simulink subsystem "controllerSSNominalReducedOrderObserver"  (R2024b)
settings: Solver=VariableStepAuto  StartTime=0.0  StopTime=10.0  RelTol=1e-3
values from neighbouring files (symbols this model uses):
  K_stateFB = place(A_c, B_c, p)    [Controller_StateSpaceDigitalController.m]
  Nu = Sol(3, :)    [Controller_StateSpaceDigitalController.m]
  Nx = Sol(1:2, :)    [Controller_StateSpaceDigitalController.m]
settings Model: Creator=Utente  LastModifiedBy=Utente

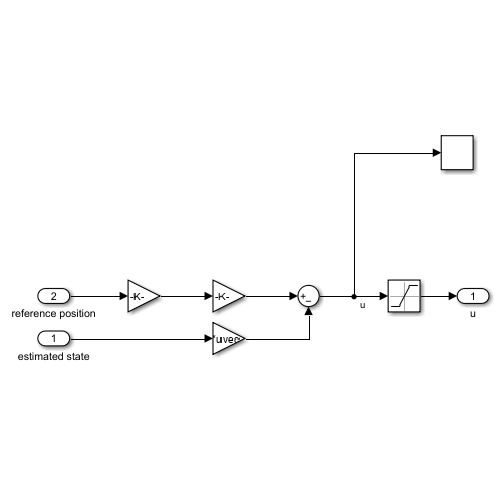
[thumbnail: Simulink's stored preview of the top-level diagram]
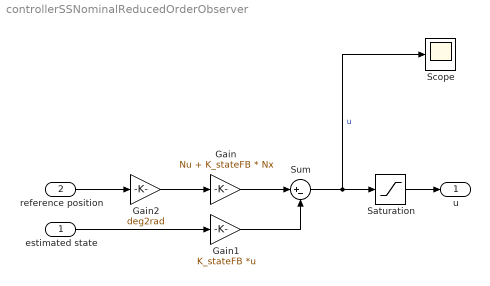
== system controllerSSNominalReducedOrderObserver ==
  estimated state : Inport
  reference position : Inport  Port=2
  Gain : Gain  Gain=Nu + K_stateFB * Nx
  Gain1 : Gain  Gain=K_stateFB  Multiplication=Matrix(K*u) (u vector)
  Gain2 : Gain  Gain=deg2rad
  Saturation : Saturate  UpperLimit=12  LowerLimit=-12
  Scope : Scope
  Sum : Sum  Inputs=|+-
  u : Outport
  wires:
  estimated state/1 -> Gain1/1
  reference position/1 -> Gain2/1
  Gain/1 -> Sum/1
  Gain1/1 -> Sum/2
  Sum/1 -> Saturation/1, Scope/1  "u"
  Gain2/1 -> Gain/1
  Saturation/1 -> u/1
